simulink model "inv_pend_delay_solo"  (Simulink 7.6)
settings: Solver=ode45  StartTime=0.0  StopTime=2  RelTol=1e-3
settings Model: Creator=mengg_000  LastModifiedBy=mengg

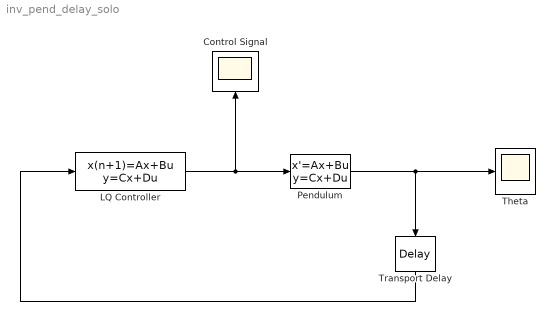
== system inv_pend_delay_solo ==
  Control Signal : Scope
      settings: TimeRange=1  YMin=1  YMax=3.5  SaveName=ry
  LQ Controller : DiscreteStateSpace  A=|  B=|  C="[-12.1798  -13.3262         0]"  D=-8.1263  X0="[0;    0;   0]"  SampleTime=0.02
      A=|
      | [0.0389   -1.5001         0;
      |     0.0828    0.3594         0;
      |   -12.1798  -13.3262         0]
      B=|
      | [ -0.4344;
      |     0.1355;
      |    -8.1263]
  "Pendulum " : StateSpace  A=[0 3.0628;32 0]  B=[2; 0]  C=[0 1.5314]  D=0  X0=[0; 0.1]
  Theta : Scope
      settings: TimeRange=1  YMin=1  YMax=3.5  SaveName=ry1
  Transport Delay : TransportDelay  DelayTime=0.01
  wires:
  "Pendulum "/1 -> Transport Delay/1, Theta/1
  Transport Delay/1 -> LQ Controller/1
  LQ Controller/1 -> "Pendulum "/1, Control Signal/1
